simulink model "vehicle_dynamics"  (R2022b)
settings: Solver=FixedStepAuto  StartTime=0.0  StopTime=10.0  FixedStep=1e-3  RelTol=1e-3
libraries: vehicle_dynamics_lib x1
settings Model: Creator=dr_pa  LastModifiedBy=dr_pa
settings DataIOCC: ExternalInput=VD_inputData.getElement('DI_p_driverTorqueRequest'),VD_inputData.getElement('DI_p_brakePedalPosition'),VD_inputData.getElement('DI_p_steeringAngle'),VD_inputData.getElement('ptCAN_AMK_ActualValues1_Left'),VD_inputData.getElement('ptCAN_AMK_ActualValues1_Right'),VD_inputData.getElement('AMKcal_n_MaxMotorSpeed'),VD_inputData.getElement('AMKcal_T_MaxMotorTorque'),VD_inputData.getElement('AMKcal_I_MaxMotorCurrent')  LoadExternalInput=on

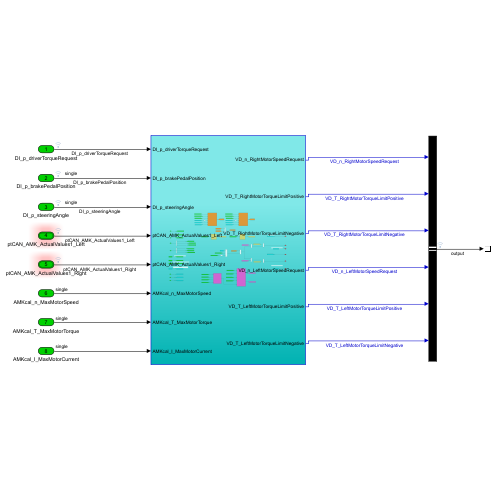
[thumbnail: Simulink's stored preview of the top-level diagram]
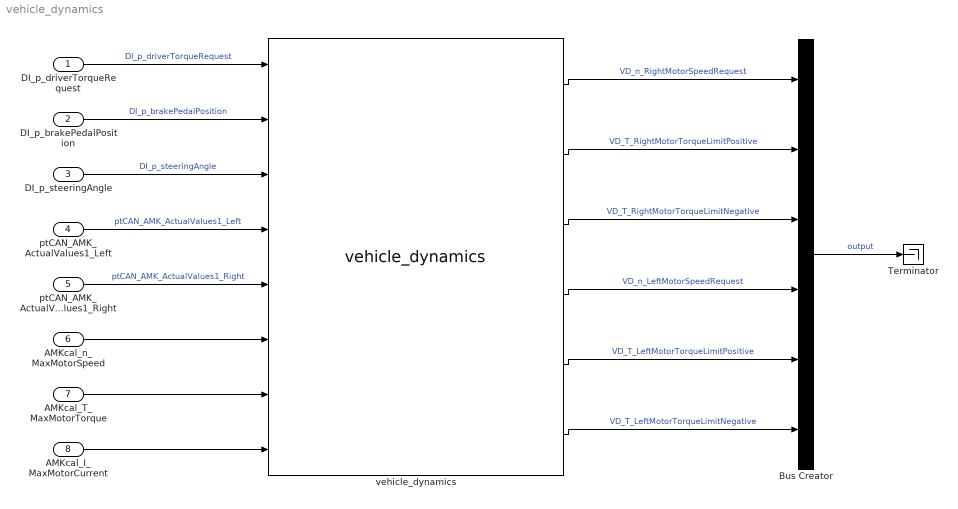
== system vehicle_dynamics ==
  DI_p_driverTorqueRequest : Inport
  DI_p_brakePedalPosition : Inport  Port=2  OutDataTypeStr=single
  DI_p_steeringAngle : Inport  Port=3  OutDataTypeStr=single
  ptCAN_AMK_ActualValues1_Left : Inport  Port=4  OutDataTypeStr=Bus: ptCAN_AMK_ActualValues1_Left_bus
  ptCAN_AMK_ActualValues1_Right : Inport  Port=5  OutDataTypeStr=Bus: ptCAN_AMK_ActualValues1_Right_bus
  AMKcal_n_MaxMotorSpeed : Inport  Port=6  OutDataTypeStr=single
  AMKcal_T_MaxMotorTorque : Inport  Port=7  OutDataTypeStr=single
  AMKcal_I_MaxMotorCurrent : Inport  Port=8  OutDataTypeStr=single
  Bus Creator : BusCreator  Inputs=6
  Terminator : Terminator
  vehicle_dynamics : vehicle_dynamics_lib/vehicle_dynamics  SystemSampleTime=-1  VariantActivationTime=update diagram  Latency=0  AutoFrameSizeCalculation=off
  wires:
  vehicle_dynamics/2 -> Bus Creator/2  "VD_T_RightMotorTorqueLimitPositive"
  vehicle_dynamics/1 -> Bus Creator/1  "VD_n_RightMotorSpeedRequest"
  vehicle_dynamics/3 -> Bus Creator/3  "VD_T_RightMotorTorqueLimitNegative"
  vehicle_dynamics/4 -> Bus Creator/4  "VD_n_LeftMotorSpeedRequest"
  vehicle_dynamics/5 -> Bus Creator/5  "VD_T_LeftMotorTorqueLimitPositive"
  Bus Creator/1 -> Terminator/1  "output"
  DI_p_driverTorqueRequest/1 -> vehicle_dynamics/1  "DI_p_driverTorqueRequest"
  DI_p_steeringAngle/1 -> vehicle_dynamics/3  "DI_p_steeringAngle"
  ptCAN_AMK_ActualValues1_Left/1 -> vehicle_dynamics/4  "ptCAN_AMK_ActualValues1_Left"
  ptCAN_AMK_ActualValues1_Right/1 -> vehicle_dynamics/5  "ptCAN_AMK_ActualValues1_Right"
  DI_p_brakePedalPosition/1 -> vehicle_dynamics/2  "DI_p_brakePedalPosition"
  vehicle_dynamics/6 -> Bus Creator/6  "VD_T_LeftMotorTorqueLimitNegative"
  AMKcal_I_MaxMotorCurrent/1 -> vehicle_dynamics/8
  AMKcal_T_MaxMotorTorque/1 -> vehicle_dynamics/7
  AMKcal_n_MaxMotorSpeed/1 -> vehicle_dynamics/6
